simulink model "Sirv1_3"  (R2023b)
settings: Solver=VariableStepAuto  StartTime=0.0  StopTime=10.0  RelTol=1e-3
undefined symbols (not defined in the file or in its folder): GOffset, Kdp, Kds, Kdt, Kdz, Kip, Kis, Kit, Kiz, Kpp, Kps, Kpt, Kpz, LSat, quadModel, USat
libraries: simulink x4, bbblueSensorLib x1
settings Model: Creator=krali  LastModifiedBy=krali

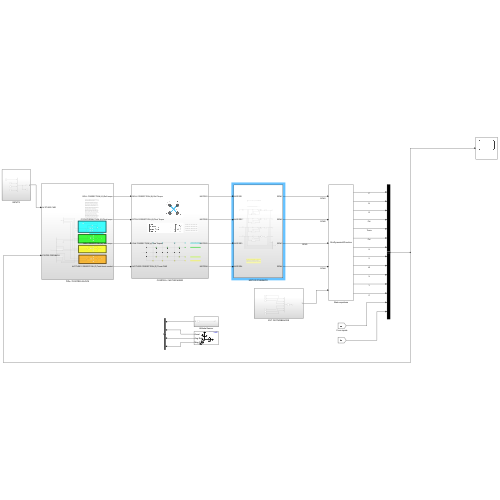
[thumbnail: Simulink's stored preview of the top-level diagram]
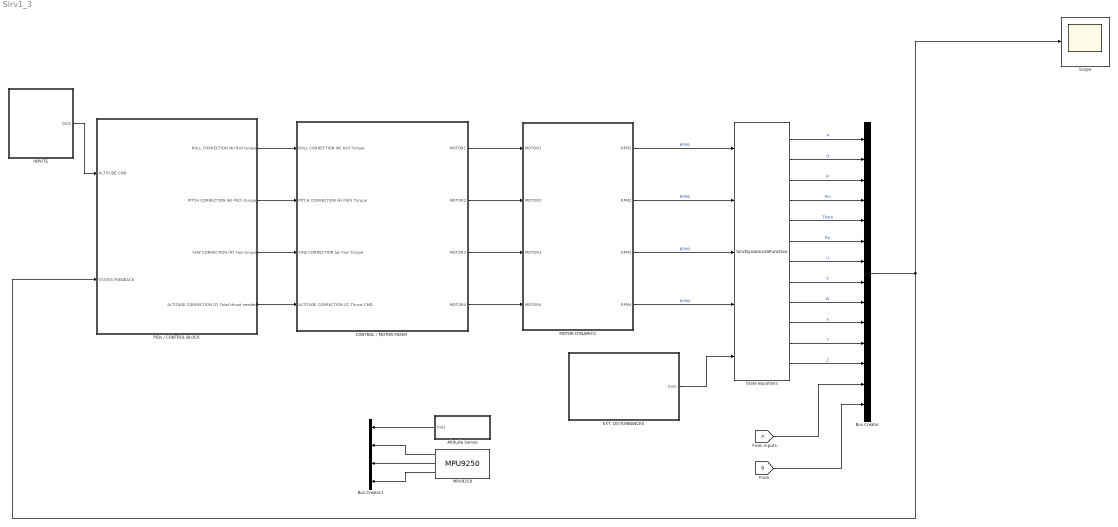
== system Sirv1_3 ==
  Altitude Sensor : Subsystem
  Bus Creator : BusCreator  Inputs=14
  Bus Creator1 : BusCreator  Inputs=4
  CONTROL / MOTOR MIXER : Subsystem
  EXT. DISTURBANCES : Subsystem
  From inputs : From  TagVisibility=global
  INPUTS : Subsystem
  MOTOR DYNAMICS : Subsystem
  MPU9250 : bbblueSensorLib/MPU9250  OperationMode=DMP  Accel=on  AngularRate=on  Ak8963Field=on  EulerAngles=off  Quat=off  AccelRange=2G  Acceldlpf=1  GyroRange=250 dps  Gyrodlpf=1  DmpOdr=200 Hz  SampleTime=0.1
  PIDs / CONTROL BLOCK : Subsystem
  Scope : Scope
  State equations : M-S-Function  FunctionName=SirvDynamicsSFunction  Parameters=quadModel, IC
  wires:
  PIDs / CONTROL BLOCK/1(ROLL CORRECTION (Φ) Roll torque) -> CONTROL / MOTOR MIXER/1(ROLL CORRECTION (Φ) Roll Torque)
  PIDs / CONTROL BLOCK/2(PITCH CORRECTION (Θ) Pitch torque) -> CONTROL / MOTOR MIXER/2(PITCH CORRECTION (θ) Pitch Torque)
  PIDs / CONTROL BLOCK/3(YAW CORRECTION (Ψ) Yaw torque) -> CONTROL / MOTOR MIXER/3(YAW CORRECTION (ψ) Yaw Torque)
  PIDs / CONTROL BLOCK/4(ALTITUDE CORRECTION (Ζ) Total thrust needed) -> CONTROL / MOTOR MIXER/4(ALTITUDE CORRECTION (Z) Thrust CMD)
  CONTROL / MOTOR MIXER/1(MOTOR1) -> MOTOR DYNAMICS/1(MOTOR1)
  CONTROL / MOTOR MIXER/2(MOTOR2) -> MOTOR DYNAMICS/2(MOTOR2)
  CONTROL / MOTOR MIXER/3(MOTOR3) -> MOTOR DYNAMICS/3(MOTOR3)
  CONTROL / MOTOR MIXER/4(MOTOR4) -> MOTOR DYNAMICS/4(MOTOR4)
  INPUTS/1(Out1) -> PIDs / CONTROL BLOCK/1(ALTITUDE CMD)
  MOTOR DYNAMICS/1(RPM1) -> State equations/1  "RPM1"
  MOTOR DYNAMICS/2(RPM2) -> State equations/2  "RPM2"
  MOTOR DYNAMICS/3(RPM3) -> State equations/3  "RPM3"
  MOTOR DYNAMICS/4(RPM4) -> State equations/4  "RPM4"
  EXT. DISTURBANCES/1(Out1) -> State equations/5
  State equations/1 -> Bus Creator/1  "P"
  State equations/2 -> Bus Creator/2  "Q"
  State equations/3 -> Bus Creator/3  "R"
  State equations/4 -> Bus Creator/4  "Phi"
  State equations/5 -> Bus Creator/5  "Theta"
  State equations/6 -> Bus Creator/6  "Psi"
  State equations/7 -> Bus Creator/7  "U"
  State equations/8 -> Bus Creator/8  "V"
  State equations/9 -> Bus Creator/9  "W"
  State equations/10 -> Bus Creator/10  "X"
  State equations/11 -> Bus Creator/11  "Y"
  State equations/12 -> Bus Creator/12  "Z"
  Bus Creator/1 -> PIDs / CONTROL BLOCK/2(STATES FEEDBACK), Scope/1
  From inputs/1 -> Bus Creator/13
  [B] -> Bus Creator/14
  MPU9250/3 -> Bus Creator1/4
  MPU9250/2 -> Bus Creator1/3
  MPU9250/1 -> Bus Creator1/2
  Altitude Sensor/1(Out1) -> Bus Creator1/1

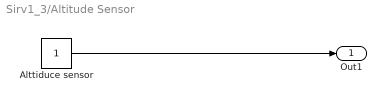
== system Sirv1_3/Altitude Sensor ==
  Alttiduce sensor : Constant
  Out1 : Outport
  wires:
  Alttiduce sensor/1 -> Out1/1

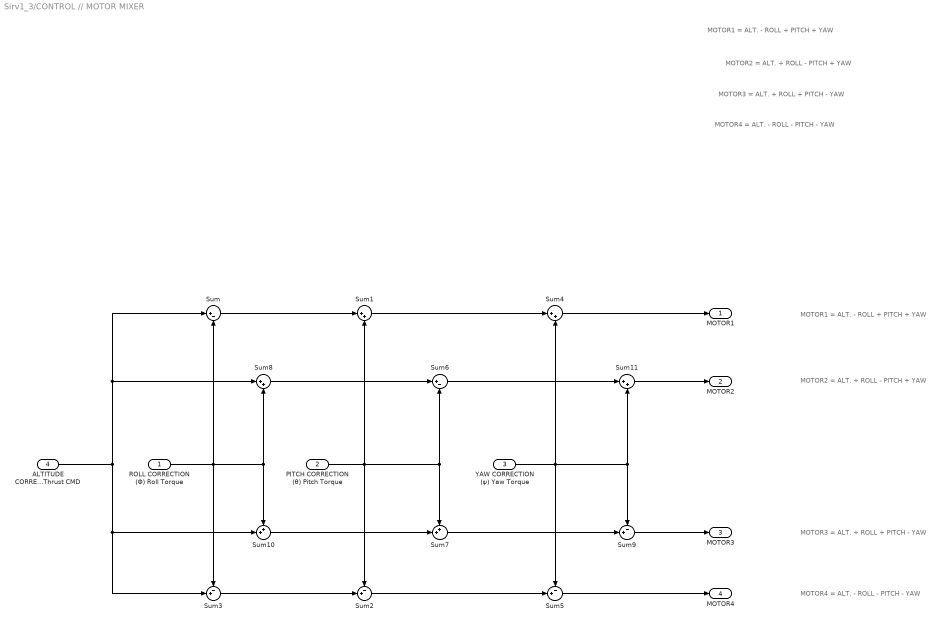
== system Sirv1_3/CONTROL // MOTOR MIXER ==
  note: MOTOR1 = ALT. - ROLL + PITCH + YAW
  note: MOTOR2 = ALT. + ROLL - PITCH + YAW
  note: MOTOR3 = ALT. + ROLL + PITCH - YAW
  note: MOTOR4 = ALT. - ROLL - PITCH - YAW
  note: MOTOR1 = ALT. - ROLL + PITCH + YAW
  note: MOTOR2 = ALT. + ROLL - PITCH + YAW
  note: MOTOR3 = ALT. + ROLL + PITCH - YAW
  note: MOTOR4 = ALT. - ROLL - PITCH - YAW
  ROLL CORRECTION (Φ) Roll Torque : Inport
  PITCH CORRECTION (θ) Pitch Torque : Inport  Port=2
  YAW CORRECTION (ψ) Yaw Torque : Inport  Port=3
  ALTITUDE CORRECTION (Z) Thrust CMD : Inport  Port=4
  Sum : Sum  Inputs=|+-
  Sum{1,4,8,11} (4 alike) : Sum  Inputs=|++
  Sum10 : Sum  Inputs=++|
  Sum{2..3,5,9} (4 alike) : Sum  Inputs=-+|
  Sum6 : Sum  Inputs=|+-
  Sum7 : Sum  Inputs=++|
  MOTOR1 : Outport
  MOTOR2 : Outport  Port=2
  MOTOR3 : Outport  Port=3
  MOTOR4 : Outport  Port=4
  wires:
  PITCH CORRECTION (θ) Pitch Torque/1 -> Sum6/2, Sum7/1, Sum2/1, Sum1/2
  ROLL CORRECTION (Φ) Roll Torque/1 -> Sum8/2, Sum10/1, Sum3/1, Sum/2
  ALTITUDE CORRECTION (Z) Thrust CMD/1 -> Sum8/1, Sum/1, Sum10/2, Sum3/2
  Sum/1 -> Sum1/1
  Sum1/1 -> Sum4/1
  Sum3/1 -> Sum2/2
  Sum2/1 -> Sum5/2
  Sum4/1 -> MOTOR1/1
  Sum5/1 -> MOTOR4/1
  Sum10/1 -> Sum7/2
  Sum7/1 -> Sum9/2
  Sum9/1 -> MOTOR3/1
  Sum8/1 -> Sum6/1
  Sum11/1 -> MOTOR2/1
  Sum6/1 -> Sum11/1
  YAW CORRECTION (ψ) Yaw Torque/1 -> Sum5/1, Sum9/1, Sum11/2, Sum4/2

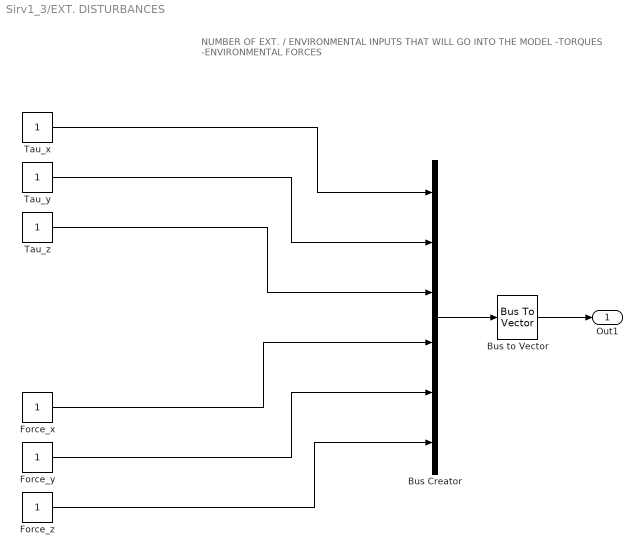
== system Sirv1_3/EXT. DISTURBANCES ==
  note: NUMBER OF EXT. / ENVIRONMENTAL INPUTS THAT WILL GO INTO THE MODEL
      | -TORQUES
      | -ENVIRONMENTAL FORCES
  Bus Creator : BusCreator  Inputs=6
  Bus to Vector : BusToVector
  Force_x : Constant
  Force_y : Constant
  Force_z : Constant
  Tau_x : Constant
  Tau_y : Constant
  Tau_z : Constant
  Out1 : Outport
  wires:
  Force_x/1 -> Bus Creator/4
  Tau_z/1 -> Bus Creator/3
  Tau_y/1 -> Bus Creator/2
  Tau_x/1 -> Bus Creator/1
  Bus Creator/1 -> Bus to Vector/1
  Bus to Vector/1 -> Out1/1
  Force_y/1 -> Bus Creator/5
  Force_z/1 -> Bus Creator/6

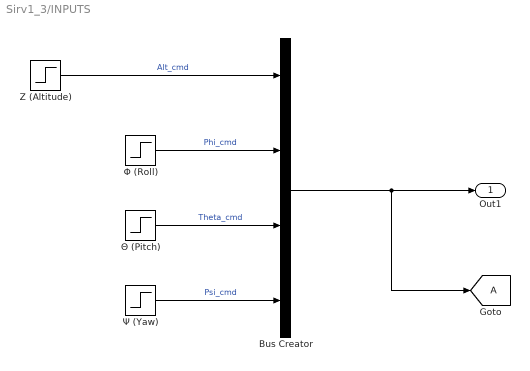
== system Sirv1_3/INPUTS ==
  Bus Creator : BusCreator  Inputs=4
  Goto : Goto  TagVisibility=global
  Z (Altitude) : Step  SampleTime=0
  Θ (Pitch) : Step  SampleTime=0
  Φ (Roll) : Step  SampleTime=0
  Ψ (Yaw) : Step  SampleTime=0
  Out1 : Outport
  wires:
  Z (Altitude)/1 -> Bus Creator/1  "Alt_cmd"
  Ψ (Yaw)/1 -> Bus Creator/4  "Psi_cmd"
  Φ (Roll)/1 -> Bus Creator/2  "Phi_cmd"
  Bus Creator/1 -> Goto/1, Out1/1
  Θ (Pitch)/1 -> Bus Creator/3  "Theta_cmd"

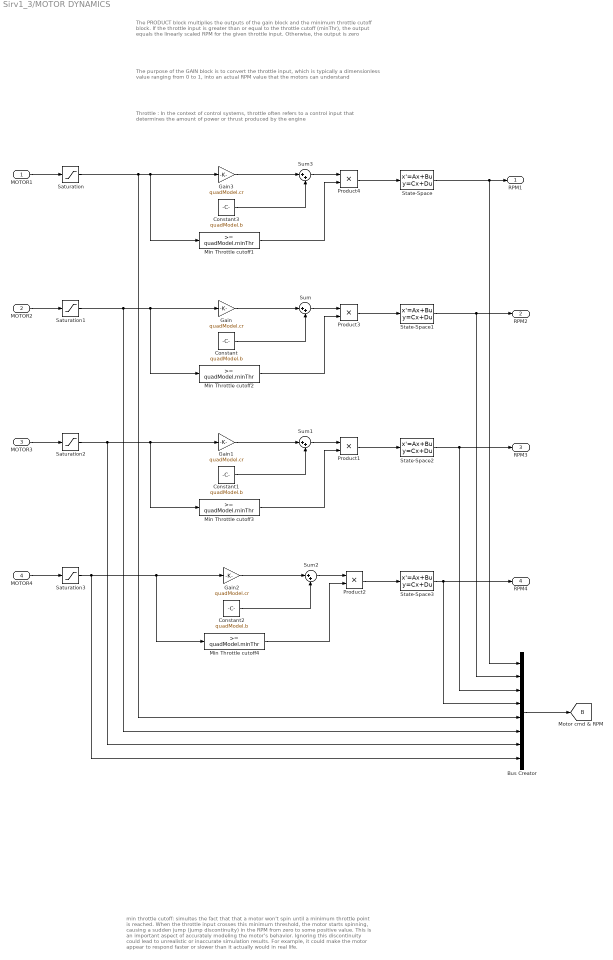
== system Sirv1_3/MOTOR DYNAMICS ==
  note: Throttle : In the context of control systems, throttle often refers to a control input that determines the amount of power or thrust produced by the engine
  note: The PRODUCT block multiplies the outputs of the gain block and the minimum throttle cutoff block. If the throttle input is greater than or equal to the throttle cutoff (minThr), the output equals the linearly scaled RPM for the given throttle input. Otherwise, the output is zero
  note: The purpose of the GAIN block is to convert the throttle input, which is typically a dimensionless value ranging from 0 to 1, into an actual RPM value that the motors can understand
  note: min throttle cutoff: simultes the fact that that a motor won't spin until a minimum throttle point is reached.
      |
      | When the throttle input crosses this minimum threshold, the motor starts spinning, causing a sudden jump (jump discontinuity) in the RPM from zero to some positive value. This is an important aspect of accurately modeling the motor’s behavior. Ignoring this discontinuity could lead to unrealistic or inaccurate simulation results. For example, it could make the motor appear to respond faster or slower than it actually would in real life.
  MOTOR1 : Inport
  MOTOR2 : Inport  Port=2
  MOTOR3 : Inport  Port=3
  MOTOR4 : Inport  Port=4
  Bus Creator : BusCreator  Inputs=8
  Constant{,1..3} (4 alike) : Constant  Value=quadModel.b
  Gain{,1..3} (4 alike) : Gain  Gain=quadModel.cr
  Min Throttle cutoff{1..4} (4 alike) : simulink/Logic and Bit Operations/Compare To Constant  relop=>=  const=quadModel.minThr  OutDataTypeStr=boolean
  Product{1..4} (4 alike) : Product
  Saturation{,1..3} (4 alike) : Saturate
  State-Space{,1..3} (4 alike) : StateSpace  InitialCondition=0
  Sum{,1..3} (4 alike) : Sum  Inputs=|++
  RPM1 : Outport
  RPM2 : Outport  Port=2
  RPM3 : Outport  Port=3
  RPM4 : Outport  Port=4
  tag scope: B=global
  wires:
  Product1/1 -> State-Space2/1
  MOTOR4/1 -> Saturation3/1
  State-Space3/1 -> Bus Creator/4, RPM4/1
  State-Space2/1 -> Bus Creator/3, RPM3/1
  MOTOR2/1 -> Saturation1/1
  State-Space/1 -> Bus Creator/1, RPM1/1
  MOTOR3/1 -> Saturation2/1
  State-Space1/1 -> Bus Creator/2, RPM2/1
  MOTOR1/1 -> Saturation/1
  Product4/1 -> State-Space/1
  Min Throttle cutoff2/1 -> Product3/2
  Saturation1/1 -> Bus Creator/6, Gain/1, Min Throttle cutoff2/1
  Sum/1 -> Product3/1
  Gain/1 -> Sum/1
  Product3/1 -> State-Space1/1
  Constant/1 -> Sum/2
  Constant1/1 -> Sum1/2
  Gain1/1 -> Sum1/1
  Sum1/1 -> Product1/1
  Saturation2/1 -> Bus Creator/7, Gain1/1, Min Throttle cutoff3/1
  Min Throttle cutoff3/1 -> Product1/2
  Constant2/1 -> Sum2/2
  Gain2/1 -> Sum2/1
  Sum2/1 -> Product2/1
  Saturation3/1 -> Bus Creator/8, Gain2/1, Min Throttle cutoff4/1
  Min Throttle cutoff4/1 -> Product2/2
  Product2/1 -> State-Space3/1
  Constant3/1 -> Sum3/2
  Gain3/1 -> Sum3/1
  Sum3/1 -> Product4/1
  Saturation/1 -> Bus Creator/5, Gain3/1, Min Throttle cutoff1/1
  Min Throttle cutoff1/1 -> Product4/2
  Bus Creator/1 -> [B]

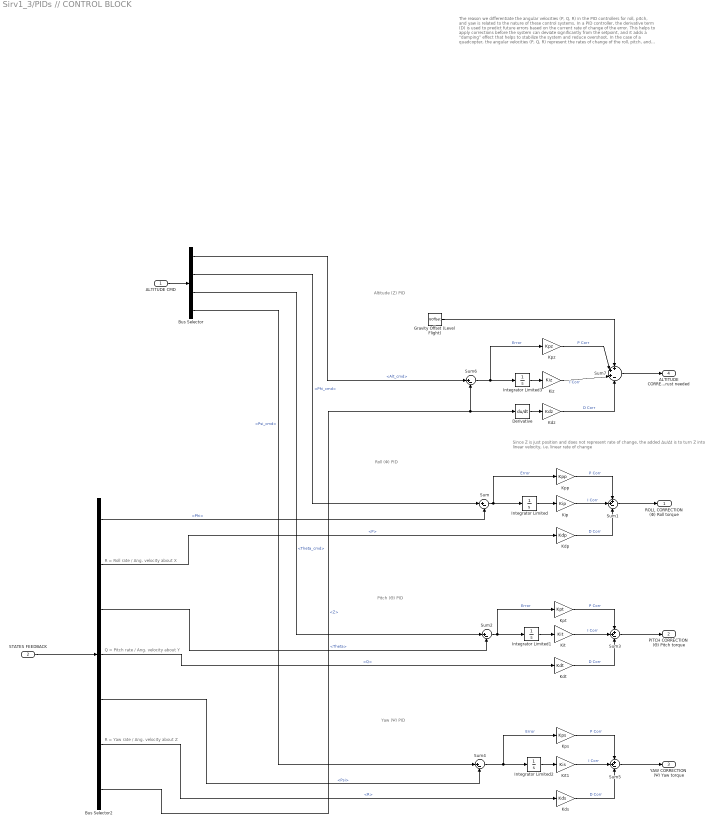
== system Sirv1_3/PIDs // CONTROL BLOCK ==
  note: Since Z is just position and does not represent rate of change, the added Δu/Δt is to turn Z into linear velocity, i.e. linear rate of change
  note: The reason we differentiate the angular velocities (P, Q, R) in the PID controllers for roll, pitch, and yaw is related to the nature of these control systems.
      | In a PID controller, the derivative term (D) is used to predict future errors based on the current rate of change of the error. This helps to apply corrections before the system can deviate significantly from the setpoint, and it adds a “damping” effect that helps to stabilize the system and reduce overshoot.
      | In the case of a quadcopter, the angular velocities (P, Q, R) represent the rates of change of the roll, pitch, and yaw angles (Phi, Theta, Psi), respectively. By differentiating these values, the PID controller can effectively “predict” changes in the roll, pitch, and yaw angles based on their current rates of change. This allows the controller to apply corrections proactively, which can result in more stable and responsive control.
      | On the other hand, the altitude PID controller differentiates the altitude (Z) because it’s directly controlling the altitude of the quadcopter, not an angular quantity. The derivative of the altitude gives the rate of change of altitude (vertical velocity), which can be used to predict future altitude errors and apply corrections accordingly.
  note: R = Yaw rate / Ang. velocity about Z
  note: Yaw (Ψ) PID
  note: Pitch (Θ) PID
  note: Roll (Φ) PID
  note: Altitude (Z) PID
  note: Q = Pitch rate / Ang. velocity about Y
  note: R = Roll rate / Ang. velocity about X
  ALTITUDE CMD : Inport
  STATES FEEDBACK : Inport  Port=2
  Bus Selector : BusSelector  OutputSignals=Alt_cmd,Phi_cmd,Theta_cmd,Psi_cmd
  Bus Selector2 : BusSelector  OutputSignals=Phi,P,Theta,Q,Psi,R,Z
  Derivative : Derivative
  Gravity Offset (Level Flight) : Constant  Value=GOffset
  Integrator Limited{,1..3} (4 alike) : Integrator  LimitOutput=on  UpperSaturationLimit=USat  LowerSaturationLimit=LSat
  Kdp : Gain  Gain=Kdp
  Kds : Gain  Gain=Kds
  Kdt : Gain  Gain=Kdt
  Kdz : Gain  Gain=Kdz
  Kip : Gain  Gain=Kip
  Kit : Gain  Gain=Kit
  Kit1 : Gain  Gain=Kis
  Kiz : Gain  Gain=Kiz
  Kpp : Gain  Gain=Kpp
  Kps : Gain  Gain=Kps
  Kpt : Gain  Gain=Kpt
  Kpz : Gain  Gain=Kpz
  Sum{,2,4,6} (4 alike) : Sum  Inputs=|+-
  Sum1 : Sum  Inputs=++-
  Sum3 : Sum  Inputs=++-
  Sum5 : Sum  Inputs=++-
  Sum7 : Sum  Inputs=+++-
  ROLL CORRECTION (Φ) Roll torque : Outport
  PITCH CORRECTION (Θ) Pitch torque : Outport  Port=2
  YAW CORRECTION (Ψ) Yaw torque : Outport  Port=3
  ALTITUDE CORRECTION (Ζ) Total thrust needed : Outport  Port=4
  wires:
  ALTITUDE CMD/1 -> Bus Selector/1
  Sum/1 -> Kpp/1, Integrator Limited/1  "Error"
  Sum1/1 -> ROLL CORRECTION (Φ) Roll torque/1
  Kip/1 -> Sum1/2  "I Corr"
  Kdp/1 -> Sum1/3  "D Corr"
  Integrator Limited/1 -> Kip/1
  Kpp/1 -> Sum1/1  "P Corr"
  STATES FEEDBACK/1 -> Bus Selector2/1
  Sum2/1 -> Integrator Limited1/1, Kpt/1  "Error"
  Sum3/1 -> PITCH CORRECTION (Θ) Pitch torque/1
  Kpt/1 -> Sum3/1  "P Corr"
  Integrator Limited1/1 -> Kit/1
  Kdt/1 -> Sum3/3  "D Corr"
  Kit/1 -> Sum3/2  "I Corr"
  Bus Selector/3 -> Sum2/1  "<Theta_cmd>"
  Bus Selector/2 -> Sum/1  "<Phi_cmd>"
  Sum5/1 -> YAW CORRECTION (Ψ) Yaw torque/1
  Bus Selector/4 -> Sum4/1  "<Psi_cmd>"
  Integrator Limited2/1 -> Kit1/1
  Kds/1 -> Sum5/3  "D Corr"
  Kps/1 -> Sum5/1  "P Corr"
  Kit1/1 -> Sum5/2  "I Corr"
  Sum4/1 -> Kps/1, Integrator Limited2/1  "Error"
  Bus Selector/1 -> Sum6/1  "<Alt_cmd>"
  Kpz/1 -> Sum7/2  "P Corr"
  Sum6/1 -> Kpz/1, Integrator Limited3/1  "Error"
  Sum7/1 -> ALTITUDE CORRECTION (Ζ) Total thrust needed/1
  Gravity Offset (Level Flight)/1 -> Sum7/1
  Kiz/1 -> Sum7/3  "I Corr"
  Kdz/1 -> Sum7/4  "D Corr"
  Derivative/1 -> Kdz/1
  Integrator Limited3/1 -> Kiz/1
  Bus Selector2/1 -> Sum/2  "<Phi>"
  Bus Selector2/2 -> Kdp/1  "<P>"
  Bus Selector2/3 -> Sum2/2  "<Theta>"
  Bus Selector2/4 -> Kdt/1  "<Q>"
  Bus Selector2/5 -> Sum4/2  "<Psi>"
  Bus Selector2/6 -> Kds/1  "<R>"
  Bus Selector2/7 -> Sum6/2, Derivative/1  "<Z>"
